simulink model "a6_3_solving_non_linear_equations"  (R2018a)
settings: Solver=VariableStepAuto  StartTime=0.0  StopTime=10.0  RelTol=1e-3
settings Model: Creator=r0x6f736f646f  LastModifiedBy=r0x6f736f646f

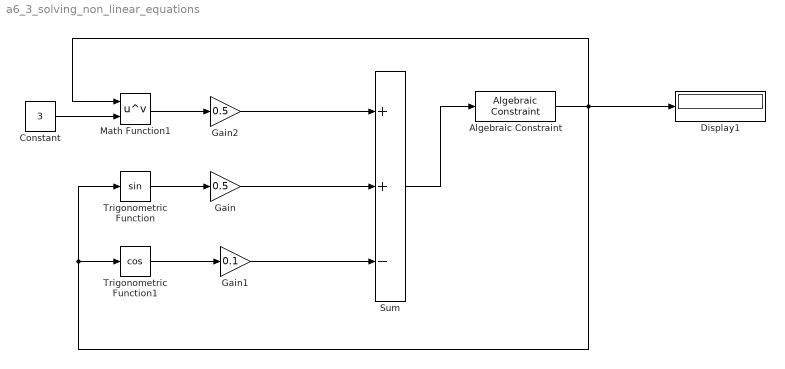
== system a6_3_solving_non_linear_equations ==
  Algebraic Constraint : AlgebraicConstraint
  Constant : Constant  Value=3
  Display1 : Display
  Gain : Gain  Gain=0.5
  Gain1 : Gain  Gain=0.1
  Gain2 : Gain  Gain=0.5
  Math Function1 : Math  Operator=pow  SaturateOnIntegerOverflow=on
  Sum : Sum  Inputs=++-
  Trigonometric Function : Trigonometry
  Trigonometric Function1 : Trigonometry  Operator=cos
  wires:
  Sum/1 -> Algebraic Constraint/1
  Gain/1 -> Sum/2
  Gain2/1 -> Sum/1
  Math Function1/1 -> Gain2/1
  Constant/1 -> Math Function1/2
  Trigonometric Function/1 -> Gain/1
  Trigonometric Function1/1 -> Gain1/1
  Algebraic Constraint/1 -> Trigonometric Function/1, Trigonometric Function1/1, Display1/1, Math Function1/1
  Gain1/1 -> Sum/3
